simulink model "useful_blocks"  (R2024b)
settings: Solver=VariableStepAuto  StartTime=0.0  StopTime=10.0  RelTol=1e-3
settings Model: Creator=s0001205361  LastModifiedBy=Franco

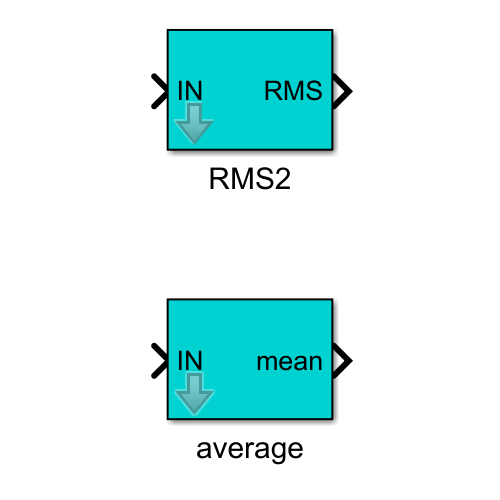
[thumbnail: Simulink's stored preview of the top-level diagram]
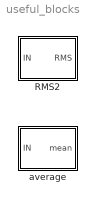
== system useful_blocks ==
  RMS2 : Subsystem  mask{period=20e-3}
      mask prompts: period "period [s]"
      mask DialogControl DescTextVar Prompt: calculates the RMS of a periodic function with period specified here
  average : Subsystem  mask{period=20}
      mask prompts: period "period [s]"

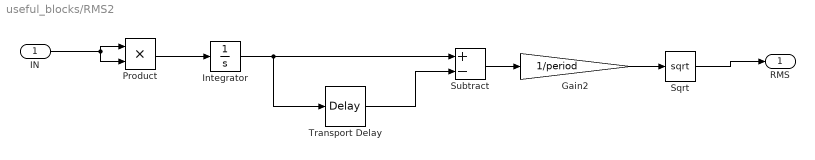
== system useful_blocks/RMS2 ==
  IN : Inport
  Gain2 : Gain  Gain=1/period
  Integrator : Integrator
  Product : Product
  Sqrt : Sqrt
  Subtract : Sum  Inputs=+-
  Transport Delay : TransportDelay  DelayTime=period
  RMS : Outport
  wires:
  Sqrt/1 -> RMS/1
  Gain2/1 -> Sqrt/1
  Product/1 -> Integrator/1
  IN/1 -> Product/2, Product/1
  Integrator/1 -> Transport Delay/1, Subtract/1
  Subtract/1 -> Gain2/1
  Transport Delay/1 -> Subtract/2

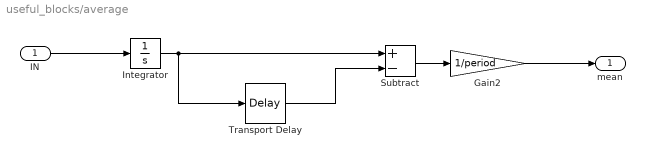
== system useful_blocks/average ==
  IN : Inport
  Gain2 : Gain  Gain=1/period
  Integrator : Integrator
  Subtract : Sum  Inputs=+-
  Transport Delay : TransportDelay  DelayTime=period
  mean : Outport
  wires:
  IN/1 -> Integrator/1
  Transport Delay/1 -> Subtract/2
  Subtract/1 -> Gain2/1
  Gain2/1 -> mean/1
  Integrator/1 -> Subtract/1, Transport Delay/1
